simulink model "ACC_System"  (R2025b)
settings: Solver=ode4  StartTime=0.0  StopTime=30  FixedStep=0.01  RelTol=1e-3
settings Model: Creator=ghazal  LastModifiedBy=ghazal

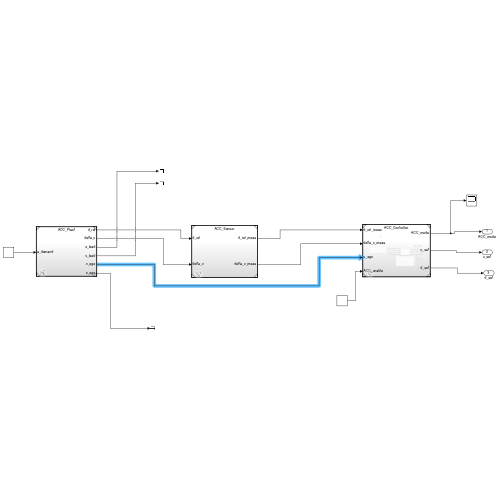
[thumbnail: Simulink's stored preview of the top-level diagram]
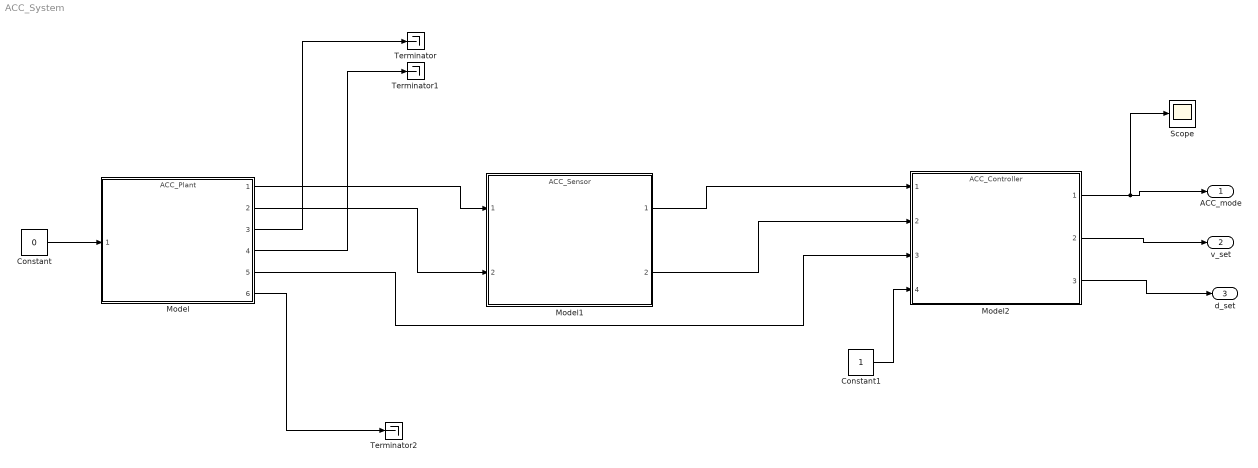
== system ACC_System ==
  Constant : Constant  Value=0
  Constant1 : Constant
  Model : ModelReference  ModelNameDialog=ACC_Plant.slx  SimulationMode=Normal  ModelReferenceVersion=1.5
  Model1 : ModelReference  ModelNameDialog=ACC_Sensor.slx  SimulationMode=Normal  ModelReferenceVersion=1.7
  Model2 : ModelReference  ModelNameDialog=ACC_Controller.slx  SimulationMode=Normal  ModelReferenceVersion=1.8
  Scope : Scope
  Terminator : Terminator
  Terminator1 : Terminator
  Terminator2 : Terminator
  ACC_mode : Outport
  v_set : Outport  Port=2
  d_set : Outport  Port=3
  wires:
  Model/1 -> Model1/1
  Model/2 -> Model1/2
  Constant/1 -> Model/1
  Model1/1 -> Model2/1
  Model1/2 -> Model2/2
  Constant1/1 -> Model2/4
  Model/5 -> Model2/3
  Model2/1 -> Scope/1, ACC_mode/1
  Model2/2 -> v_set/1
  Model2/3 -> d_set/1
  Model/3 -> Terminator/1
  Model/4 -> Terminator1/1
  Model/6 -> Terminator2/1
